simulink model "GFLIB_ControllerPIrAW_BAM_FLT"  (Simulink 8.3)
settings: Solver=ode45  StartTime=0.0  StopTime=10.0  RelTol=1e-3
undefined symbols (not defined in the file): fltCC1, fltCC2
settings Model: Creator=B17364  LastModifiedBy=B17364
settings DataIOCC: SignalLoggingSaveFormat=Dataset
settings DebuggingCC: UnderspecifiedInitializationDetection=Simplified  StateNameClashWarn=none
settings GRTTargetCC: CombineOutputUpdateFcns=on  GRTInterface=off

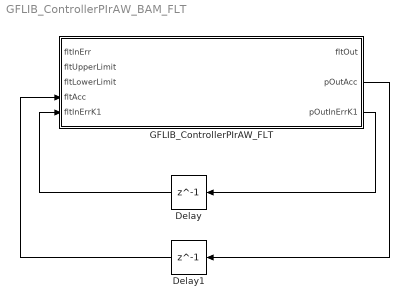
== system GFLIB_ControllerPIrAW_BAM_FLT ==
  Delay : Delay  DelayLength=1  InitialCondition=0
  Delay1 : Delay  DelayLength=1  InitialCondition=0
  GFLIB_ControllerPIrAW_FLT : Subsystem  mask(GFLIB_ControllerPIrAW_FLT){fltCC1=fltCC1, fltCC2=fltCC2}
      mask help: Bit accurate model of reccurent form PI controller with anti-windup. All parameters as well as input and output are single precison floating point numbers.
      mask init:
      | pos = get_param(gcb, 'Position');width = pos(3) - pos(1); height = pos(4) - pos(2);tX=width/2;tY=height*0.9;
      mask Display: color('black');port_label('input',1,'fltInErr');port_label('input',2,'fltUpperLimit');port_label('input',3,'fltLowerLimit');port_label('input',4,'fltAcc');port_label('input',5,'fltInErrK1');port_label('output',1,'fltOut');port_label('output',2,'pOutAcc');port_label('output',3,'pOutInErrK1');color('black');disp('GFLIB_ControllerPIrAW_FLT');color('blue');text(tX,tY, 'BAM', 'horizontalAlignment', 'center');
  wires:
  GFLIB_ControllerPIrAW_FLT/3(pOutInErrK1) -> Delay/1
  GFLIB_ControllerPIrAW_FLT/2(pOutAcc) -> Delay1/1
  Delay/1 -> GFLIB_ControllerPIrAW_FLT/5(fltInErrK1)
  Delay1/1 -> GFLIB_ControllerPIrAW_FLT/4(fltAcc)

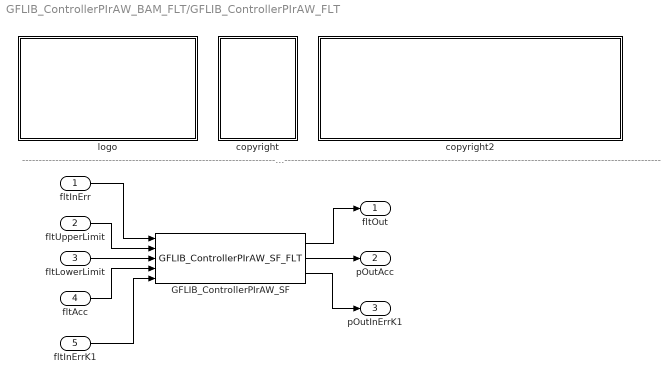
== system GFLIB_ControllerPIrAW_BAM_FLT/GFLIB_ControllerPIrAW_FLT ==
  note: ---------------------------------------------------------------------------------------------------------------------------------------------------------------------------------------------------
  fltInErr : Inport
  fltUpperLimit : Inport  Port=2
  fltLowerLimit : Inport  Port=3
  fltAcc : Inport  Port=4
  fltInErrK1 : Inport  Port=5
  GFLIB_ControllerPIrAW_SF : S-Function  FunctionName=GFLIB_ControllerPIrAW_SF_FLT  Parameters=fltCC1,fltCC2  EnableBusSupport=off
  copyright : Subsystem
      mask Display: text(10,90,'FILE:');text(10,75,'DESRIPTION:');text(10,60,'COPYRIGHT:');text(10,45,'VERSION:');text(10,30,'DATE:')
  copyright2 : Subsystem
      mask Display: text(10,90,'GFLIB_ControllerPIrAW_BAM_FLT.mdl');text(10,75,'Recurrent form of a standard PI controller with implemented anti-windup functionality .');text(10,60,'Freescale');text(10,45,'0.1');text(10,30,'12-Jun-2015');
  logo : Subsystem
      mask Display: image(imread('logo.jpg'))
  fltOut : Outport
  pOutAcc : Outport  Port=2
  pOutInErrK1 : Outport  Port=3
  wires:
  fltInErr/1 -> GFLIB_ControllerPIrAW_SF/1
  fltUpperLimit/1 -> GFLIB_ControllerPIrAW_SF/2
  fltLowerLimit/1 -> GFLIB_ControllerPIrAW_SF/3
  fltAcc/1 -> GFLIB_ControllerPIrAW_SF/4
  fltInErrK1/1 -> GFLIB_ControllerPIrAW_SF/5
  GFLIB_ControllerPIrAW_SF/1 -> fltOut/1
  GFLIB_ControllerPIrAW_SF/2 -> pOutAcc/1
  GFLIB_ControllerPIrAW_SF/3 -> pOutInErrK1/1

== system GFLIB_ControllerPIrAW_BAM_FLT/GFLIB_ControllerPIrAW_FLT/copyright ==

== system GFLIB_ControllerPIrAW_BAM_FLT/GFLIB_ControllerPIrAW_FLT/copyright2 ==

== system GFLIB_ControllerPIrAW_BAM_FLT/GFLIB_ControllerPIrAW_FLT/logo ==
